simulink subsystem "Electromechanical_SubSystem"  (R2021a)
settings: Solver=VariableStepAuto  StartTime=0.0  StopTime=10.0  RelTol=1e-3
undefined symbols (not defined in the file): body, Fv1, g, g1q, gbox, M11q, M22q, mot, ua2tau1, wheel, x0_q, x0_qdot
settings Model: Creator=utente-A  LastModifiedBy=utente-A

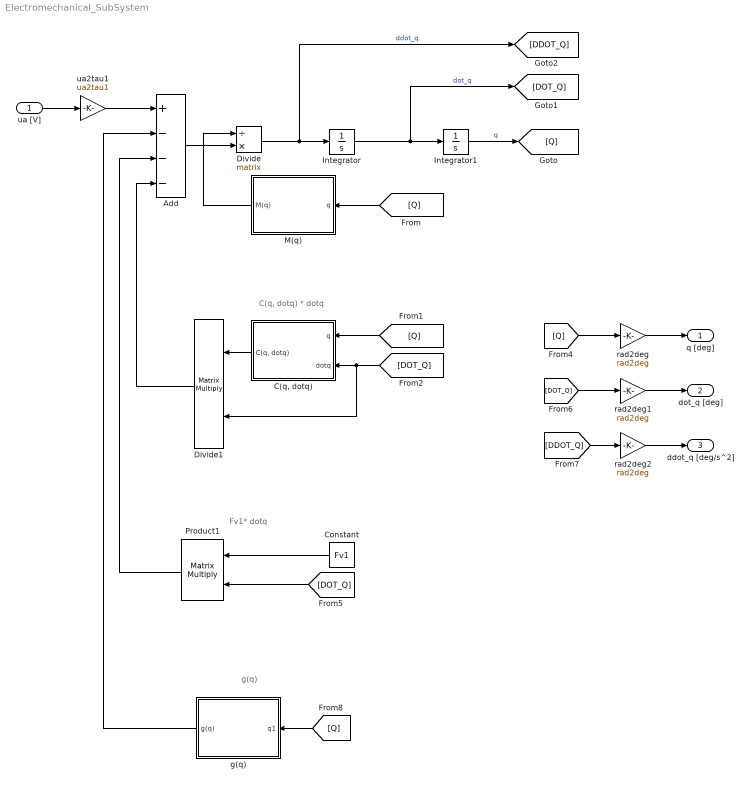
== system Electromechanical_SubSystem ==
  note: C(q, dotq) * dotq
  note: Fv1* dotq
  note: g(q)
  ua [V] : Inport
  Add : Sum  Inputs=+---
  "C(q, dotq)" : Subsystem
  Constant : Constant  Value=Fv1
  Divide : Product  Inputs=/*  Multiplication=Matrix(*)
  Divide1 : Product  Inputs=**  Multiplication=Matrix(*)
  Integrator : Integrator  InitialCondition=x0_qdot
  Integrator1 : Integrator  InitialCondition=x0_q
  M(q) : Subsystem
  Product1 : Product  Multiplication=Matrix(*)
  g(q) : Subsystem
  rad2deg : Gain  Gain=rad2deg
  rad2deg1 : Gain  Gain=rad2deg
  rad2deg2 : Gain  Gain=rad2deg
  ua2tau1 : Gain  Gain=ua2tau1
  q [deg] : Outport
  dot_q [deg] : Outport  Port=2
  ddot_q [deg/s^2] : Outport  Port=3
  wires:
  [Q] -> "C(q, dotq)"/1(q)
  ua2tau1/1 -> Add/1
  Integrator/1 -> Integrator1/1, [DOT_Q]  "dot_q"
  Divide/1 -> Integrator/1, [DDOT_Q]  "ddot_q"
  Integrator1/1 -> [Q]  "q"
  ua [V]/1 -> ua2tau1/1
  [Q] -> M(q)/1(q)
  Divide1/1 -> Add/4
  "C(q, dotq)"/1("C(q, dotq)") -> Divide1/1
  rad2deg1/1 -> dot_q [deg]/1
  [DOT_Q] -> rad2deg1/1
  [DOT_Q] -> Divide1/2, "C(q, dotq)"/2(dotq)
  [Q] -> rad2deg/1
  rad2deg2/1 -> ddot_q [deg/s^2]/1
  [DDOT_Q] -> rad2deg2/1
  rad2deg/1 -> q [deg]/1
  [Q] -> g(q)/1(q1)
  Product1/1 -> Add/3
  [DOT_Q] -> Product1/2
  Constant/1 -> Product1/1
  g(q)/1(g(q)) -> Add/2
  M(q)/1(M(q)) -> Divide/1
  Add/1 -> Divide/2

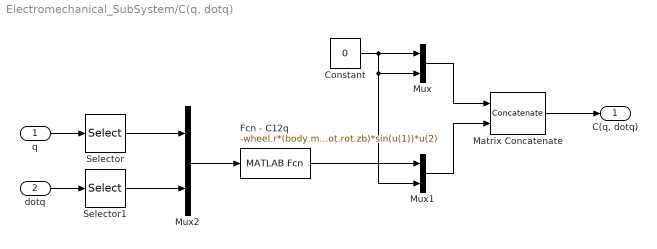
== system Electromechanical_SubSystem/C(q, dotq) ==
  q : Inport
  dotq : Inport  Port=2
  Constant : Constant  Value=0
  Fcn - C12q : MATLABFcn  MATLABFcn=-wheel.r*(body.m*body.zb + 2*mot.rot.m*mot.rot.zb)*sin(u(1))*u(2)
  Matrix Concatenate : Concatenate  Mode=Multidimensional array  ConcatenateDimension=2
  Mux : Mux  Inputs=2
  Mux1 : Mux  Inputs=2
  Mux2 : Mux  Inputs=2
  Selector : Selector  InputPortWidth=2  IndexOptions=Starting index (dialog)  Indices=2  OutputSizes=1
  Selector1 : Selector  InputPortWidth=2  IndexOptions=Starting index (dialog)  Indices=2  OutputSizes=1
  "C(q, dotq)" : Outport
  wires:
  Fcn - C12q/1 -> Mux1/1
  Mux2/1 -> Fcn - C12q/1
  Selector1/1 -> Mux2/2
  Selector/1 -> Mux2/1
  dotq/1 -> Selector1/1
  Matrix Concatenate/1 -> "C(q, dotq)"/1
  Mux1/1 -> Matrix Concatenate/2
  Constant/1 -> Mux1/2, Mux/2, Mux/1
  Mux/1 -> Matrix Concatenate/1
  q/1 -> Selector/1

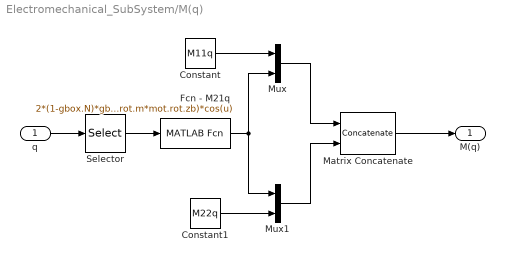
== system Electromechanical_SubSystem/M(q) ==
  q : Inport
  Constant : Constant  Value=M11q
  Constant1 : Constant  Value=M22q
  Fcn - M21q : MATLABFcn  MATLABFcn=2*(1-gbox.N)*gbox.N*mot.rot.Iyy + wheel.r*(body.zb*body.m + 2*mot.rot.m*mot.rot.zb)*cos(u)
  Matrix Concatenate : Concatenate  Mode=Multidimensional array  ConcatenateDimension=2
  Mux : Mux  Inputs=2
  Mux1 : Mux  Inputs=2
  Selector : Selector  InputPortWidth=2  IndexOptions=Starting index (dialog)  Indices=2  OutputSizes=1
  M(q) : Outport
  wires:
  Matrix Concatenate/1 -> M(q)/1
  Mux1/1 -> Matrix Concatenate/2
  Fcn - M21q/1 -> Mux1/1, Mux/2
  Constant1/1 -> Mux1/2
  Constant/1 -> Mux/1
  Mux/1 -> Matrix Concatenate/1
  Selector/1 -> Fcn - M21q/1
  q/1 -> Selector/1

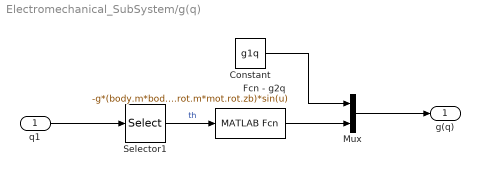
== system Electromechanical_SubSystem/g(q) ==
  q1 : Inport
  Constant : Constant  Value=g1q
  Fcn - g2q : MATLABFcn  MATLABFcn=-g*(body.m*body.zb + 2*mot.rot.m*mot.rot.zb)*sin(u)
  Mux : Mux  Inputs=2
  Selector1 : Selector  InputPortWidth=2  IndexOptions=Index vector (dialog)  Indices=[2]  OutputSizes=1
  g(q) : Outport
  wires:
  q1/1 -> Selector1/1
  Constant/1 -> Mux/1
  Selector1/1 -> Fcn - g2q/1  "th"
  Mux/1 -> g(q)/1
  Fcn - g2q/1 -> Mux/2
